simulink model "simulink223"  (R2020b)
settings: Solver=VariableStepAuto  StartTime=0.0  StopTime=1  RelTol=1e-3
libraries: simulink x2
settings Model: Creator=Nikita  LastModifiedBy=Nikita

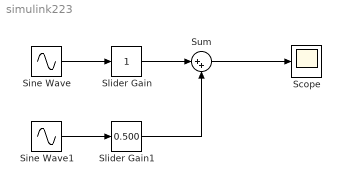
== system simulink223 ==
  Scope : Scope
  Sine Wave : Sin  SineType=Sample based  Frequency=2*pi*2  Samples=48  SampleTime=1/48000
  Sine Wave1 : Sin  SineType=Sample based  Frequency=2*pi*2  Samples=24  SampleTime=1/48000
  Slider Gain : simulink/Math Operations/Slider Gain  gain=1  low=0  high=2
  Slider Gain1 : simulink/Math Operations/Slider Gain  gain=0.500  low=0  high=1
  Sum : Sum  Inputs=|++
  wires:
  Slider Gain/1 -> Sum/1
  Sine Wave/1 -> Slider Gain/1
  Sum/1 -> Scope/1
  Sine Wave1/1 -> Slider Gain1/1
  Slider Gain1/1 -> Sum/2
